simulink model "NIMBY"  (R2023a)
settings: Solver=VariableStepAuto  StartTime=0.0  StopTime=runtime  RelTol=1e-3
values from neighbouring files (symbols this model uses):
  DroneMass = 0.1    [NimbyCode.m]
  Dx = 1.5    [NimbyCode.m]
  Dy = 1.5    [NimbyCode.m]
  Dz = 2.5    [NimbyCode.m]
  escapeMargin = 1    [NimbyCode.m]
  Gravity = 9.81    [NimbyCode.m]
  InitialWPS = [InitialPosition; 0 0 -10]    [NimbyCode.m]
  Ix = 0    [NimbyCode.m]
  Iy = 0    [NimbyCode.m]
  Iz = 0    [NimbyCode.m]
  Nx = 1.25*10    (= 12.5)    [NimbyCode.m]
  Ny = 1.25*10    (= 12.5)    [NimbyCode.m]
  Nz = 1.25*14.4947065605712    (= 18.1183832007)    [NimbyCode.m]
  obstacleHeight = 15    [NimbyCode.m]
  obstaclePos = [5 5 0;5 25 0; 25 25 0; 25 5 0]    [NimbyCode.m]
  obstacleWidth = 5    [NimbyCode.m]
  Px = 6    [NimbyCode.m]
  Py = 6    [NimbyCode.m]
  Pz = 6.5    [NimbyCode.m]
  UAVSampleTime = 0.01    [NimbyCode.m]
libraries: slpidlib x6, dspsrcs4 x4, uavsimlib x4, robotcorelib x2, uavalgslib x2
settings Model: PacingRate=1000  Creator=JoshJ  LastModifiedBy=JoshJ
settings DebuggingCC: ParameterOverflowMsg=none  ParameterPrecisionLossMsg=none

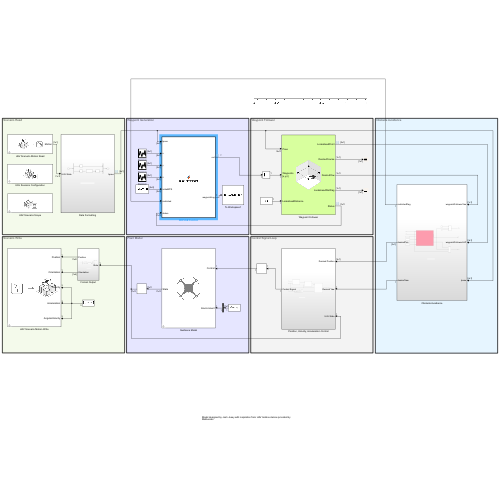
[thumbnail: Simulink's stored preview of the top-level diagram]
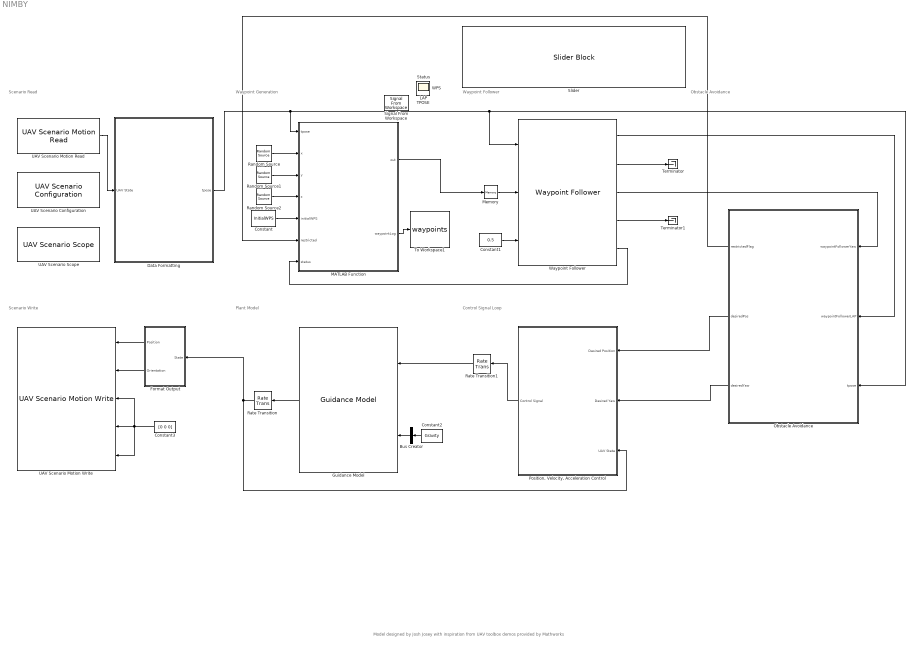
== system NIMBY ==
  note: Model designed by Josh Josey with inspiration from UAV toolbox demos provided by Mathworks
  note: Obstacle Avoidance
  note: Control Signal Loop
  note: Waypoint Follower
  note: Scenario Read
  note: Plant Model
  note: Scenario Write
  note: Waypoint Generation
  Bus Creator : BusCreator  Inputs=1  OutDataTypeStr=Bus: uavGuidanceEnvironmentBus  NonVirtualBus=on
      settings: InheritFromInputs=off
  Constant : Constant  Value=InitialWPS
  Constant1 : Constant  Value=0.5
  Constant2 : Constant  Value=Gravity  OutDataTypeStr=double
  Constant3 : Constant  Value=[0 0 0]
  Data Formatting : Subsystem
  Format Output : Subsystem
  Guidance Model : uavalgslib/Guidance Model  ModelType=MultirotorGuidance  SpecifiedDataType=double  SimulateUsing=Code generation  InitialWorldPositionMultirotor=InitialPosition'  InitialWorldVelocityMultirotor=[0; 0; 0]  InitialEulerZYXMultirotor=[0; 0; 0]  InitialBodyAngularRateRPYMultirotor=[0; 0; 0]  InitialThrustMultirotor=0  InitialNorthFixedWing=0  InitialEastFixedWing=0  InitialHeightFixedWing=0  InitialAirSpeedFixedWing=0  InitialHeadingAngleFixedWing=0  InitialFlightPathAngleFixedWing=0  InitialRollAngleFixedWing=0  InitialRollAngleRateFixedWing=0  PDRollMultirotor=[3402.97,116.67]  PDPitchMultirotor=[3402.97, 116.67]  PYawRateMultirotor=1950  PThrustMultirotor=3900  MassMultirotor=0.1  PHeightFixedWing=3.9  PHeadingAngleFixedWing=3.9  PFlightPathAngleFixedWing=39  PDRollFixedWing=[3402.97, 116.67]  PAirSpeedFixedWing=1  FlightPathAngleLimitsFixedWing=[-pi/2, pi/2]  StateBusName='uavGuidanceStateBus'  ControlBusName='uavGuidanceControlBus'  EnvironmentBusName='uavGuidanceEnvironmentBus'  DataType=double
  MATLAB Function : MATLAB Function  TreatAsAtomicUnit=on  SystemSampleTime=UAVSampleTime
  Memory : Memory
  Obstacle Avoidance : Subsystem
  "Position, Velocity, Acceleration Control" : Subsystem
  Random Source : dspsrcs4/Random Source  SrcType=Uniform  NormMethod=Ziggurat  CltLength=12  MinVal=0  MaxVal=30  MeanVal=0  VarVal=1  RepMode=Not repeatable  rawSeed=1  IsInherit=off  SampMode=Discrete  SampTime=UAVSampleTime  SampFrame=2  DataType=Double  OutComplex=Real  OutputFrames=off
  Random Source1 : dspsrcs4/Random Source  SrcType=Uniform  NormMethod=Ziggurat  CltLength=12  MinVal=0  MaxVal=30  MeanVal=0  VarVal=1  RepMode=Not repeatable  rawSeed=1  IsInherit=off  SampMode=Discrete  SampTime=UAVSampleTime  SampFrame=2  DataType=Double  OutComplex=Real  OutputFrames=off
  Random Source2 : dspsrcs4/Random Source  SrcType=Uniform  NormMethod=Ziggurat  CltLength=12  MinVal=5  MaxVal=20  MeanVal=0  VarVal=1  RepMode=Not repeatable  rawSeed=1  IsInherit=off  SampMode=Discrete  SampTime=UAVSampleTime  SampFrame=2  DataType=Double  OutComplex=Real  OutputFrames=off
  Rate Transition : RateTransition  OutPortSampleTime=UAVSampleTime
  Rate Transition1 : RateTransition  OutPortSampleTime=UAVSampleTime
  Slider : SliderBlock  LabelPosition=Hide  ScaleMax=1  TickInterval=.2
  Terminator : Terminator
  Terminator1 : Terminator
  To Workspace1 : ToWorkspace  VariableName=waypoints  SampleTime=-1
  UAV Scenario Configuration : uavsimlib/UAV Scenario Configuration  Priority=-1  UAVScenarioObject=Scenario  SampleTime=0.1  UpdateParam=false  SensorMotionBusName='SensorMotionBus'  PlatformMotionBusName='PlatformMotionBus'  ScenarioMotionBusName='ScenarioMotionBus'  ScenarioMotionSignalName='ScenarioMotions'
  UAV Scenario Motion Read : uavsimlib/UAV Scenario Motion Read  Priority=1  EntityName='UAV'  ReferenceFrame=NED
  UAV Scenario Motion Write : uavsimlib/UAV Scenario Motion Write  Priority=0  PlatName='UAV'  ReferenceFrame=NED
  UAV Scenario Scope : uavsimlib/UAV Scenario Scope  Priority=1  SensorNameTable={}  SampleTime=0.1
  Waypoint Follower : uavalgslib/Waypoint Follower  UAVType=multirotor  StartFrom=first  TransitionRadiusSource=internal  TransitionRadius=.1  MinLookaheadDistance=.2  YawInput=off  ShowCrossTrackErrorOutput=off  ShowStatusOutput=on  SimulateUsing=Code generation
  LAP : Scope
  Signal From Workspace : dspsrcs4/Signal From Workspace  IOType=siggen  X=1:10  Ts=1  nsamps=1  OutputAfterFinalValue=Setting to zero  ignoreOrWarnInputAndFrameLengths=off  OutputFrames=on
      settings: LibrarySourceBlock=|
      | dspgenerators/Signal From
      | Workspace
  Status : Scope
  TPOSE : Scope
  WPS : Scope
  wires:
  UAV Scenario Motion Read/1 -> Data Formatting/1(UAV State)
  Data Formatting/1(tpose) -> MATLAB Function/1(tpose), Obstacle Avoidance/3(tpose), Waypoint Follower/1
  Constant1/1 -> Waypoint Follower/3
  Waypoint Follower/2 -> Terminator/1
  Waypoint Follower/4 -> Terminator1/1
  Guidance Model/1 -> Rate Transition/1
  Rate Transition/1 -> Format Output/1(State), "Position, Velocity, Acceleration Control"/3(UAV State)
  Bus Creator/1 -> Guidance Model/2
  Constant2/1 -> Bus Creator/1
  Rate Transition1/1 -> Guidance Model/1
  Constant3/1 -> UAV Scenario Motion Write/5, UAV Scenario Motion Write/3, UAV Scenario Motion Write/4
  Format Output/2(Orientation) -> UAV Scenario Motion Write/2
  Format Output/1(Position) -> UAV Scenario Motion Write/1
  Waypoint Follower/5 -> MATLAB Function/7(status)
  Memory/1 -> Waypoint Follower/2
  MATLAB Function/1(out) -> Memory/1
  "Position, Velocity, Acceleration Control"/1(Control Signal) -> Rate Transition1/1
  Waypoint Follower/1 -> Obstacle Avoidance/2(waypointFollowerLAP)
  Waypoint Follower/3 -> Obstacle Avoidance/1(waypointFollowerYaw)
  Obstacle Avoidance/1(restrictedFlag) -> MATLAB Function/6(restricted)
  Obstacle Avoidance/2(desiredPos) -> "Position, Velocity, Acceleration Control"/1(Desired Position)
  Obstacle Avoidance/3(desiredYaw) -> "Position, Velocity, Acceleration Control"/2(Desired Yaw)
  MATLAB Function/2(waypointLog) -> To Workspace1/1
  Constant/1 -> MATLAB Function/5(initialWPS)
  Random Source2/1 -> MATLAB Function/4(z)
  Random Source1/1 -> MATLAB Function/3(y)
  Random Source/1 -> MATLAB Function/2(x)

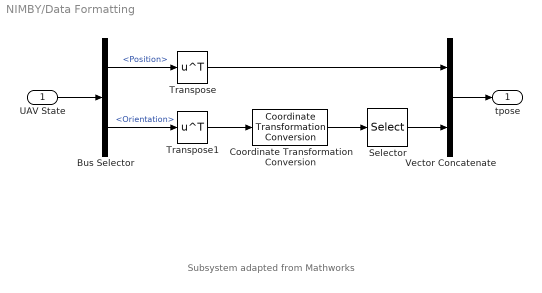
== system NIMBY/Data Formatting ==
  note: Subsystem adapted from Mathworks
  UAV State : Inport
  Bus Selector : BusSelector  OutputSignals=Position,Orientation
  Coordinate Transformation Conversion : robotcorelib/Coordinate Transformation Conversion  InputRepresentation=Quaternion  InputEulerSequence=ZYX  ShowTrVecInputPort=on  OutputRepresentation=Euler Angles  OutputEulerSequence=ZYX  ShowTrVecOutputPort=on  SimulateUsing=Interpreted execution
      settings: LibrarySourceBlock=navlib/Utilities/Coordinate Transformation Conversion
  Selector : Selector  InputPortWidth=3  IndexOptions=Index vector (dialog)  Indices=[1]  OutputSizes=1
  Transpose : Math  Operator=transpose
  Transpose1 : Math  Operator=transpose
  Vector Concatenate : Concatenate
  tpose : Outport
  wires:
  UAV State/1 -> Bus Selector/1
  Transpose1/1 -> Coordinate Transformation Conversion/1
  Bus Selector/1 -> Transpose/1  "<Position>"
  Bus Selector/2 -> Transpose1/1  "<Orientation>"
  Vector Concatenate/1 -> tpose/1
  Transpose/1 -> Vector Concatenate/1
  Coordinate Transformation Conversion/1 -> Selector/1
  Selector/1 -> Vector Concatenate/2

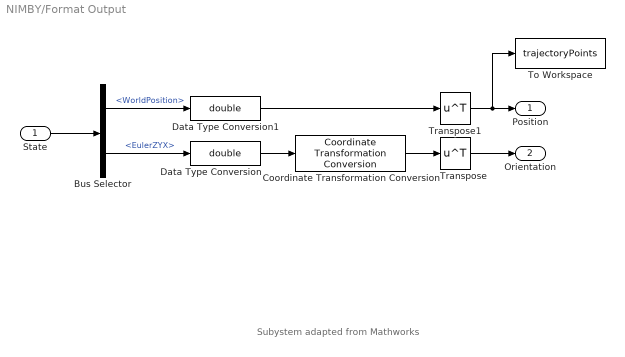
== system NIMBY/Format Output ==
  note: Subystem adapted from Mathworks
  State : Inport
  Bus Selector : BusSelector  OutputSignals=WorldPosition,EulerZYX
  Coordinate Transformation Conversion : robotcorelib/Coordinate Transformation Conversion  InputRepresentation=Euler Angles  InputEulerSequence=ZYX  ShowTrVecInputPort=on  OutputRepresentation=Quaternion  OutputEulerSequence=ZYX  ShowTrVecOutputPort=on  SimulateUsing=Code generation
      settings: LibrarySourceBlock=navlib/Utilities/Coordinate Transformation Conversion
  Data Type Conversion : DataTypeConversion  OutDataTypeStr=double  SaturateOnIntegerOverflow=off  RndMeth=Floor
  Data Type Conversion1 : DataTypeConversion  OutDataTypeStr=double  SaturateOnIntegerOverflow=off  RndMeth=Floor
  To Workspace : ToWorkspace  VariableName=trajectoryPoints  SampleTime=-1
  Transpose : Math  Operator=transpose
  Transpose1 : Math  Operator=transpose
  Position : Outport
  Orientation : Outport  Port=2
  wires:
  State/1 -> Bus Selector/1
  Bus Selector/1 -> Data Type Conversion1/1  "<WorldPosition>"
  Bus Selector/2 -> Data Type Conversion/1  "<EulerZYX>"
  Data Type Conversion/1 -> Coordinate Transformation Conversion/1
  Transpose/1 -> Orientation/1
  Coordinate Transformation Conversion/1 -> Transpose/1
  Data Type Conversion1/1 -> Transpose1/1
  Transpose1/1 -> To Workspace/1, Position/1

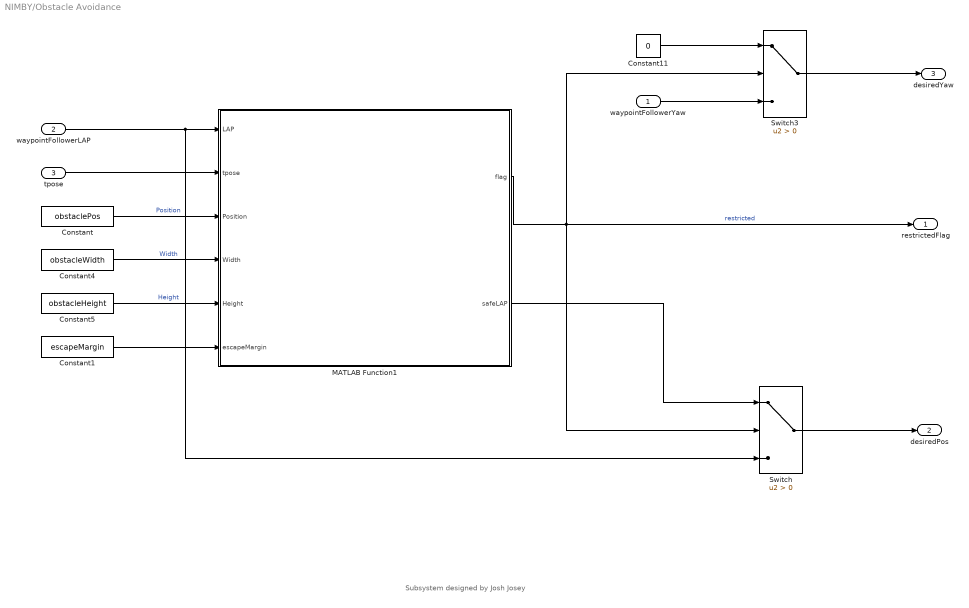
== system NIMBY/Obstacle Avoidance ==
  note: Subsystem designed by Josh Josey
  waypointFollowerYaw : Inport
  waypointFollowerLAP : Inport  Port=2
  tpose : Inport  Port=3
  Constant : Constant  Value=obstaclePos
  Constant1 : Constant  Value=escapeMargin
  Constant11 : Constant  Value=0
  Constant4 : Constant  Value=obstacleWidth
  Constant5 : Constant  Value=obstacleHeight
  MATLAB Function1 : MATLAB Function  TreatAsAtomicUnit=on
  Switch : Switch  Criteria=u2 > Threshold  SaturateOnIntegerOverflow=off  InputSameDT=off
  Switch3 : Switch  Criteria=u2 > Threshold  SaturateOnIntegerOverflow=off  InputSameDT=off
  restrictedFlag : Outport
  desiredPos : Outport  Port=2
  desiredYaw : Outport  Port=3
  wires:
  tpose/1 -> MATLAB Function1/2(tpose)
  Constant4/1 -> MATLAB Function1/4(Width)  "Width"
  Constant11/1 -> Switch3/1
  MATLAB Function1/1(flag) -> Switch3/2, Switch/2, restrictedFlag/1  "restricted"
  Constant5/1 -> MATLAB Function1/5(Height)  "Height"
  Constant/1 -> MATLAB Function1/3(Position)  "Position"
  Switch3/1 -> desiredYaw/1
  waypointFollowerLAP/1 -> Switch/3, MATLAB Function1/1(LAP)
  Switch/1 -> desiredPos/1
  waypointFollowerYaw/1 -> Switch3/3
  MATLAB Function1/2(safeLAP) -> Switch/1
  Constant1/1 -> MATLAB Function1/6(escapeMargin)

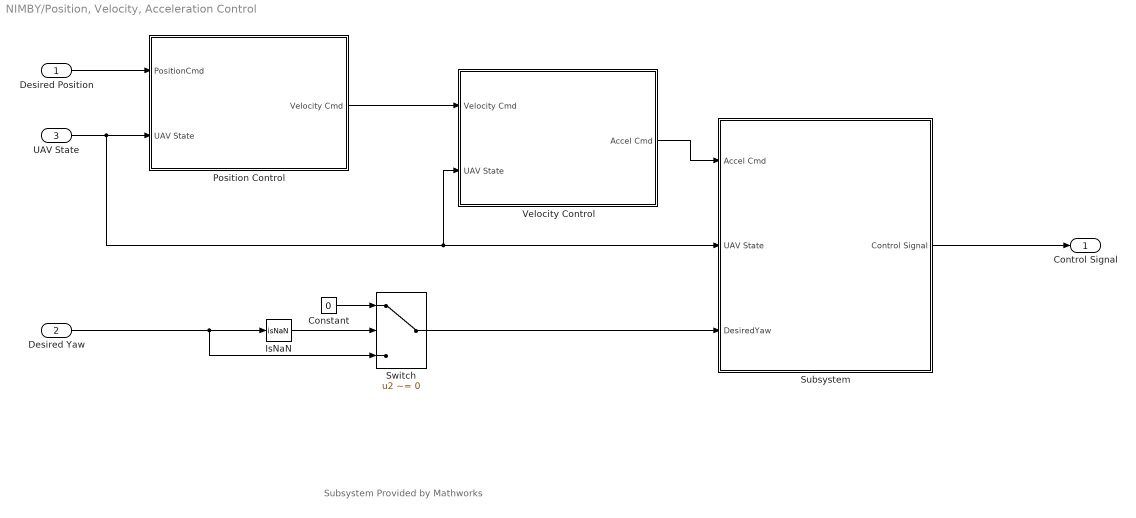
== system NIMBY/Position, Velocity, Acceleration Control ==
  note: Subsystem Provided by Mathworks
  Desired Position : Inport
  Desired Yaw : Inport  Port=2
  UAV State : Inport  Port=3
  Constant : Constant  Value=0  OutDataTypeStr=Inherit: Inherit via back propagation
  IsNaN : RelationalOperator  Operator=isNaN  OutDataTypeStr=boolean  RndMeth=Simplest  InputSameDT=off
  Position Control : Subsystem
  Subsystem : Subsystem
  Switch : Switch  Criteria=u2 ~= 0  SaturateOnIntegerOverflow=off  InputSameDT=off
  Velocity Control : Subsystem
  Control Signal : Outport
  wires:
  Desired Yaw/1 -> Switch/3, IsNaN/1
  UAV State/1 -> Subsystem/2(UAV State), Velocity Control/2(UAV State), Position Control/2(UAV State)
  Desired Position/1 -> Position Control/1(PositionCmd)
  Position Control/1(Velocity Cmd) -> Velocity Control/1(Velocity Cmd)
  Subsystem/1(Control Signal) -> Control Signal/1
  Velocity Control/1(Accel Cmd) -> Subsystem/1(Accel Cmd)
  IsNaN/1 -> Switch/2
  Constant/1 -> Switch/1
  Switch/1 -> Subsystem/3(DesiredYaw)

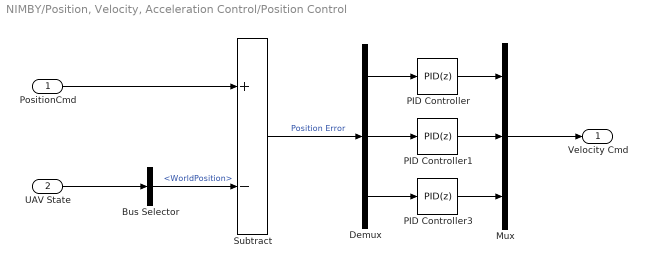
== system NIMBY/Position, Velocity, Acceleration Control/Position Control ==
  PositionCmd : Inport
  UAV State : Inport  Port=2
  Bus Selector : BusSelector  OutputSignals=WorldPosition
  Demux : Demux  Outputs=3
  Mux : Mux  Inputs=3
  PID Controller : slpidlib/PID Controller  Controller=PID  Form=Parallel  TimeDomain=Discrete-time  UseExternalTs=off  SampleTime=-1  IntegratorMethod=Forward Euler  FilterMethod=Forward Euler  ControllerParametersSource=internal  P=Px  I=Ix  UseKiTs=off  D=Dx  N=Nx  UseFilter=on  TunerSelectOption=Transfer Function Based (PID Tuner App)  InitialConditionSource=internal  InitialConditionForIntegrator=0  InitialConditionForFilter=0  DifferentiatorICPrevScaledInput=0  ExternalReset=none  TrackingMode=off  Kt=1  LimitOutput=on  SatLimitsSource=internal  UpperSaturationLimit=3  LowerSaturationLimit=-3  LinearizeAsGain=on  AntiWindupMode=clamping  Kb=1  LimitIntegrator=off  UpperIntegratorSaturationLimit=inf  LowerIntegratorSaturationLimit=-inf  POutMin=[]  POutMax=[]  IOutMin=[]  IOutMax=[]  DOutMin=[]  DOutMax=[]  NOutMin=[]  NOutMax=[]  SumOutMin=[]  SumOutMax=[]  SaturationOutMin=[]  SaturationOutMax=[]  PParamMin=[]  PParamMax=[]  IParamMin=[]  IParamMax=[]  DParamMin=[]  DParamMax=[]  NParamMin=[]  NParamMax=[]  KbParamMin=[]  KbParamMax=[]  KtParamMin=[]  KtParamMax=[]  KbOutMin=[]  KbOutMax=[]  KtOutMin=[]  KtOutMax=[]  IntegratorOutMin=[]  IntegratorOutMax=[]  FilterOutMin=[]  FilterOutMax=[]  SumI1OutMin=[]  SumI1OutMax=[]  SumI2OutMin=[]  SumI2OutMax=[]  SumI3OutMin=[]  SumI3OutMax=[]  SumI4OutMin=[]  SumI4OutMax=[]  SumDOutMin=[]  SumDOutMax=[]  DifferentiatorOutMin=[]  DifferentiatorOutMax=[]  FilterDiffOutCoefMin=[]  FilterDiffOutCoefMax=[]  ReciprocalOutMin=[]  ReciprocalOutMax=[]  SumDenOutMin=[]  SumDenOutMax=[]  SumNumOutMin=[]  SumNumOutMax=[]  DivideOutMin=[]  DivideOutMax=[]  UdiffTsProdOutMin=[]  UdiffTsProdOutMax=[]  NTsProdOutMin=[]  NTsProdOutMax=[]  UintegralTsProdOutMin=[]  UintegralTsProdOutMax=[]  UngainTsProdOutMin=[]  UngainTsProdOutMax=[]  ClampingZeroOutDataTypeStr=Inherit: Inherit via back propagation  ClampingZeroOutMin=[]  ClampingZeroOutMax=[]  FilterDenConstantOutDataTypeStr=Inherit: Inherit via back propagation  FilterDenConstantOutMin=[]  FilterDenConstantOutMax=[]  PCopyOutDataTypeStr=Inherit: Inherit via back propagation  PCopyOutMin=[]  PCopyOutMax=[]  NCopyOutDataTypeStr=Inherit: Inherit via back propagation  NCopyOutMin=[]  NCopyOutMax=[]  IntegratorContinuousStateAttributes=''  IntegratorStateMustResolveToSignalObject=off  IntegratorRTWStateStorageClass=Auto  FilterContinuousStateAttributes=''  FilterStateMustResolveToSignalObject=off  FilterRTWStateStorageClass=Auto  ParallelPVariant=InternalParameters  IdealPVariant=Disabled  IVariant=InternalParameters  DVariant=InternalParameters  IntegratorVariant=Discrete  SatVariant=Enabled  AWVariant=DiscClampingParallel  PCopyVariant=Disabled  TRVariant=Disabled  FdbkBlocksVariant=Forward  IdealPFdbkVariant=Disabled  SatFdbkVariant=Disabled  DerivativeFilterVariant=ForwardEulerFilter  NVariant=InternalParameters  NCopyVariant=Disabled  FilterICVariant=InternalICsFilter  IntegratorICVariant=InternalICs  ExternalResetVariant=Disabled  TRSumVariant=Passthrough  SumFdbkVariant=Disabled  SumVariant=Sum_PID  TsampFilterVariant=InternalTs  TsampNgainVariant=Passthrough  TsampIntegralVariant=Disabled_SignalSpec  ExternalSaturationOutDataTypeStr=Inherit: Same as second input
  PID Controller1 : slpidlib/PID Controller  Controller=PID  Form=Parallel  TimeDomain=Discrete-time  UseExternalTs=off  SampleTime=-1  IntegratorMethod=Forward Euler  FilterMethod=Forward Euler  ControllerParametersSource=internal  P=Py  I=Iy  UseKiTs=off  D=Dy  N=Ny  UseFilter=on  TunerSelectOption=Transfer Function Based (PID Tuner App)  InitialConditionSource=internal  InitialConditionForIntegrator=0  InitialConditionForFilter=0  DifferentiatorICPrevScaledInput=0  ExternalReset=none  TrackingMode=off  Kt=1  LimitOutput=on  SatLimitsSource=internal  UpperSaturationLimit=3  LowerSaturationLimit=-3  LinearizeAsGain=on  AntiWindupMode=clamping  Kb=1  LimitIntegrator=off  UpperIntegratorSaturationLimit=inf  LowerIntegratorSaturationLimit=-inf  POutMin=[]  POutMax=[]  IOutMin=[]  IOutMax=[]  DOutMin=[]  DOutMax=[]  NOutMin=[]  NOutMax=[]  SumOutMin=[]  SumOutMax=[]  SaturationOutMin=[]  SaturationOutMax=[]  PParamMin=[]  PParamMax=[]  IParamMin=[]  IParamMax=[]  DParamMin=[]  DParamMax=[]  NParamMin=[]  NParamMax=[]  KbParamMin=[]  KbParamMax=[]  KtParamMin=[]  KtParamMax=[]  KbOutMin=[]  KbOutMax=[]  KtOutMin=[]  KtOutMax=[]  IntegratorOutMin=[]  IntegratorOutMax=[]  FilterOutMin=[]  FilterOutMax=[]  SumI1OutMin=[]  SumI1OutMax=[]  SumI2OutMin=[]  SumI2OutMax=[]  SumI3OutMin=[]  SumI3OutMax=[]  SumI4OutMin=[]  SumI4OutMax=[]  SumDOutMin=[]  SumDOutMax=[]  DifferentiatorOutMin=[]  DifferentiatorOutMax=[]  FilterDiffOutCoefMin=[]  FilterDiffOutCoefMax=[]  ReciprocalOutMin=[]  ReciprocalOutMax=[]  SumDenOutMin=[]  SumDenOutMax=[]  SumNumOutMin=[]  SumNumOutMax=[]  DivideOutMin=[]  DivideOutMax=[]  UdiffTsProdOutMin=[]  UdiffTsProdOutMax=[]  NTsProdOutMin=[]  NTsProdOutMax=[]  UintegralTsProdOutMin=[]  UintegralTsProdOutMax=[]  UngainTsProdOutMin=[]  UngainTsProdOutMax=[]  ClampingZeroOutDataTypeStr=Inherit: Inherit via back propagation  ClampingZeroOutMin=[]  ClampingZeroOutMax=[]  FilterDenConstantOutDataTypeStr=Inherit: Inherit via back propagation  FilterDenConstantOutMin=[]  FilterDenConstantOutMax=[]  PCopyOutDataTypeStr=Inherit: Inherit via back propagation  PCopyOutMin=[]  PCopyOutMax=[]  NCopyOutDataTypeStr=Inherit: Inherit via back propagation  NCopyOutMin=[]  NCopyOutMax=[]  IntegratorContinuousStateAttributes=''  IntegratorStateMustResolveToSignalObject=off  IntegratorRTWStateStorageClass=Auto  FilterContinuousStateAttributes=''  FilterStateMustResolveToSignalObject=off  FilterRTWStateStorageClass=Auto  ParallelPVariant=InternalParameters  IdealPVariant=Disabled  IVariant=InternalParameters  DVariant=InternalParameters  IntegratorVariant=Discrete  SatVariant=Enabled  AWVariant=DiscClampingParallel  PCopyVariant=Disabled  TRVariant=Disabled  FdbkBlocksVariant=Forward  IdealPFdbkVariant=Disabled  SatFdbkVariant=Disabled  DerivativeFilterVariant=ForwardEulerFilter  NVariant=InternalParameters  NCopyVariant=Disabled  FilterICVariant=InternalICsFilter  IntegratorICVariant=InternalICs  ExternalResetVariant=Disabled  TRSumVariant=Passthrough  SumFdbkVariant=Disabled  SumVariant=Sum_PID  TsampFilterVariant=InternalTs  TsampNgainVariant=Passthrough  TsampIntegralVariant=Disabled_SignalSpec  ExternalSaturationOutDataTypeStr=Inherit: Same as second input
  PID Controller3 : slpidlib/PID Controller  Controller=PID  Form=Parallel  TimeDomain=Discrete-time  UseExternalTs=off  SampleTime=-1  IntegratorMethod=Forward Euler  FilterMethod=Forward Euler  ControllerParametersSource=internal  P=Pz  I=Iz  UseKiTs=off  D=Dz  N=Nz  UseFilter=on  TunerSelectOption=Transfer Function Based (PID Tuner App)  InitialConditionSource=internal  InitialConditionForIntegrator=0  InitialConditionForFilter=0  DifferentiatorICPrevScaledInput=0  ExternalReset=none  TrackingMode=off  Kt=1  LimitOutput=on  SatLimitsSource=internal  UpperSaturationLimit=3  LowerSaturationLimit=-3  LinearizeAsGain=on  AntiWindupMode=clamping  Kb=1  LimitIntegrator=off  UpperIntegratorSaturationLimit=inf  LowerIntegratorSaturationLimit=-inf  POutMin=[]  POutMax=[]  IOutMin=[]  IOutMax=[]  DOutMin=[]  DOutMax=[]  NOutMin=[]  NOutMax=[]  SumOutMin=[]  SumOutMax=[]  SaturationOutMin=[]  SaturationOutMax=[]  PParamMin=[]  PParamMax=[]  IParamMin=[]  IParamMax=[]  DParamMin=[]  DParamMax=[]  NParamMin=[]  NParamMax=[]  KbParamMin=[]  KbParamMax=[]  KtParamMin=[]  KtParamMax=[]  KbOutMin=[]  KbOutMax=[]  KtOutMin=[]  KtOutMax=[]  IntegratorOutMin=[]  IntegratorOutMax=[]  FilterOutMin=[]  FilterOutMax=[]  SumI1OutMin=[]  SumI1OutMax=[]  SumI2OutMin=[]  SumI2OutMax=[]  SumI3OutMin=[]  SumI3OutMax=[]  SumI4OutMin=[]  SumI4OutMax=[]  SumDOutMin=[]  SumDOutMax=[]  DifferentiatorOutMin=[]  DifferentiatorOutMax=[]  FilterDiffOutCoefMin=[]  FilterDiffOutCoefMax=[]  ReciprocalOutMin=[]  ReciprocalOutMax=[]  SumDenOutMin=[]  SumDenOutMax=[]  SumNumOutMin=[]  SumNumOutMax=[]  DivideOutMin=[]  DivideOutMax=[]  UdiffTsProdOutMin=[]  UdiffTsProdOutMax=[]  NTsProdOutMin=[]  NTsProdOutMax=[]  UintegralTsProdOutMin=[]  UintegralTsProdOutMax=[]  UngainTsProdOutMin=[]  UngainTsProdOutMax=[]  ClampingZeroOutDataTypeStr=Inherit: Inherit via back propagation  ClampingZeroOutMin=[]  ClampingZeroOutMax=[]  FilterDenConstantOutDataTypeStr=Inherit: Inherit via back propagation  FilterDenConstantOutMin=[]  FilterDenConstantOutMax=[]  PCopyOutDataTypeStr=Inherit: Inherit via back propagation  PCopyOutMin=[]  PCopyOutMax=[]  NCopyOutDataTypeStr=Inherit: Inherit via back propagation  NCopyOutMin=[]  NCopyOutMax=[]  IntegratorContinuousStateAttributes=''  IntegratorStateMustResolveToSignalObject=off  IntegratorRTWStateStorageClass=Auto  FilterContinuousStateAttributes=''  FilterStateMustResolveToSignalObject=off  FilterRTWStateStorageClass=Auto  ParallelPVariant=InternalParameters  IdealPVariant=Disabled  IVariant=InternalParameters  DVariant=InternalParameters  IntegratorVariant=Discrete  SatVariant=Enabled  AWVariant=DiscClampingParallel  PCopyVariant=Disabled  TRVariant=Disabled  FdbkBlocksVariant=Forward  IdealPFdbkVariant=Disabled  SatFdbkVariant=Disabled  DerivativeFilterVariant=ForwardEulerFilter  NVariant=InternalParameters  NCopyVariant=Disabled  FilterICVariant=InternalICsFilter  IntegratorICVariant=InternalICs  ExternalResetVariant=Disabled  TRSumVariant=Passthrough  SumFdbkVariant=Disabled  SumVariant=Sum_PID  TsampFilterVariant=InternalTs  TsampNgainVariant=Passthrough  TsampIntegralVariant=Disabled_SignalSpec  ExternalSaturationOutDataTypeStr=Inherit: Same as second input
  Subtract : Sum  Inputs=+-
  Velocity Cmd : Outport
  wires:
  UAV State/1 -> Bus Selector/1
  PositionCmd/1 -> Subtract/1
  Bus Selector/1 -> Subtract/2  "<WorldPosition>"
  Subtract/1 -> Demux/1  "Position Error"
  Demux/1 -> PID Controller/1
  Demux/2 -> PID Controller1/1
  Demux/3 -> PID Controller3/1
  PID Controller3/1 -> Mux/3
  Mux/1 -> Velocity Cmd/1
  PID Controller1/1 -> Mux/2
  PID Controller/1 -> Mux/1

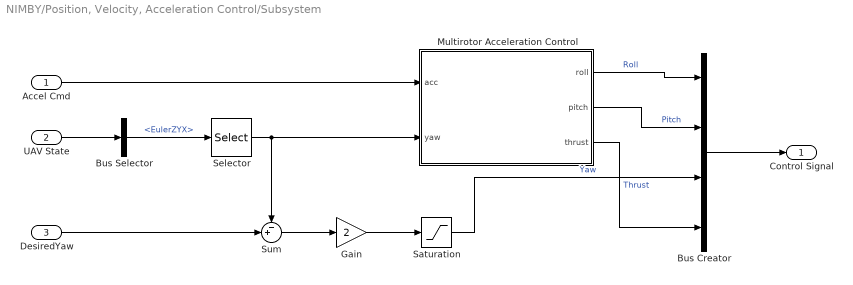
== system NIMBY/Position, Velocity, Acceleration Control/Subsystem ==
  Accel Cmd : Inport
  UAV State : Inport  Port=2
  DesiredYaw : Inport  Port=3
  Bus Creator : BusCreator  Inputs=4  OutDataTypeStr=Bus: uavGuidanceControlBus  NonVirtualBus=on
      settings: InheritFromInputs=off
  Bus Selector : BusSelector  OutputSignals=EulerZYX
  Gain : Gain  Gain=2
  Multirotor Acceleration Control : MATLAB Function  TreatAsAtomicUnit=on
  Saturation : Saturate
  Selector : Selector  InputPortWidth=3  IndexOptions=Index vector (dialog)  Indices=1  OutputSizes=1
  Sum : Sum  Inputs=-+|
  Control Signal : Outport
  wires:
  Multirotor Acceleration Control/2(pitch) -> Bus Creator/2  "Pitch"
  Multirotor Acceleration Control/1(roll) -> Bus Creator/1  "Roll"
  Bus Creator/1 -> Control Signal/1
  Multirotor Acceleration Control/3(thrust) -> Bus Creator/4  "Thrust"
  Accel Cmd/1 -> Multirotor Acceleration Control/1(acc)
  UAV State/1 -> Bus Selector/1
  Bus Selector/1 -> Selector/1  "<EulerZYX>"
  Selector/1 -> Sum/1, Multirotor Acceleration Control/2(yaw)
  DesiredYaw/1 -> Sum/2
  Sum/1 -> Gain/1
  Gain/1 -> Saturation/1
  Saturation/1 -> Bus Creator/3  "Yaw"

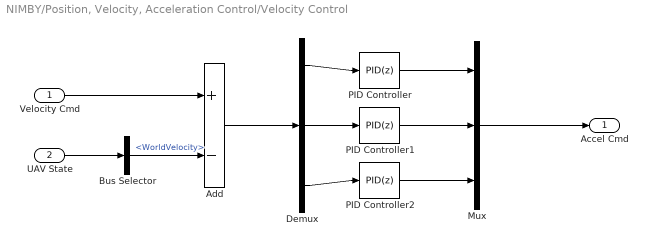
== system NIMBY/Position, Velocity, Acceleration Control/Velocity Control ==
  Velocity Cmd : Inport
  UAV State : Inport  Port=2
  Add : Sum  Inputs=+-
  Bus Selector : BusSelector  OutputSignals=WorldVelocity
  Demux : Demux  Outputs=3
  Mux : Mux  Inputs=3
  PID Controller : slpidlib/PID Controller  Controller=PID  Form=Parallel  TimeDomain=Discrete-time  UseExternalTs=off  SampleTime=-1  IntegratorMethod=Forward Euler  FilterMethod=Forward Euler  ControllerParametersSource=internal  P=Px  I=Ix  UseKiTs=off  D=Dx  N=Nx  UseFilter=on  TunerSelectOption=Transfer Function Based (PID Tuner App)  InitialConditionSource=internal  InitialConditionForIntegrator=0  InitialConditionForFilter=0  DifferentiatorICPrevScaledInput=0  ExternalReset=none  TrackingMode=off  Kt=1  LimitOutput=on  SatLimitsSource=internal  UpperSaturationLimit=3  LowerSaturationLimit=-3  LinearizeAsGain=on  AntiWindupMode=clamping  Kb=1  LimitIntegrator=off  UpperIntegratorSaturationLimit=inf  LowerIntegratorSaturationLimit=-inf  POutMin=[]  POutMax=[]  IOutMin=[]  IOutMax=[]  DOutMin=[]  DOutMax=[]  NOutMin=[]  NOutMax=[]  SumOutMin=[]  SumOutMax=[]  SaturationOutMin=[]  SaturationOutMax=[]  PParamMin=[]  PParamMax=[]  IParamMin=[]  IParamMax=[]  DParamMin=[]  DParamMax=[]  NParamMin=[]  NParamMax=[]  KbParamMin=[]  KbParamMax=[]  KtParamMin=[]  KtParamMax=[]  KbOutMin=[]  KbOutMax=[]  KtOutMin=[]  KtOutMax=[]  IntegratorOutMin=[]  IntegratorOutMax=[]  FilterOutMin=[]  FilterOutMax=[]  SumI1OutMin=[]  SumI1OutMax=[]  SumI2OutMin=[]  SumI2OutMax=[]  SumI3OutMin=[]  SumI3OutMax=[]  SumI4OutMin=[]  SumI4OutMax=[]  SumDOutMin=[]  SumDOutMax=[]  DifferentiatorOutMin=[]  DifferentiatorOutMax=[]  FilterDiffOutCoefMin=[]  FilterDiffOutCoefMax=[]  ReciprocalOutMin=[]  ReciprocalOutMax=[]  SumDenOutMin=[]  SumDenOutMax=[]  SumNumOutMin=[]  SumNumOutMax=[]  DivideOutMin=[]  DivideOutMax=[]  UdiffTsProdOutMin=[]  UdiffTsProdOutMax=[]  NTsProdOutMin=[]  NTsProdOutMax=[]  UintegralTsProdOutMin=[]  UintegralTsProdOutMax=[]  UngainTsProdOutMin=[]  UngainTsProdOutMax=[]  ClampingZeroOutDataTypeStr=Inherit: Inherit via back propagation  ClampingZeroOutMin=[]  ClampingZeroOutMax=[]  FilterDenConstantOutDataTypeStr=Inherit: Inherit via back propagation  FilterDenConstantOutMin=[]  FilterDenConstantOutMax=[]  PCopyOutDataTypeStr=Inherit: Inherit via back propagation  PCopyOutMin=[]  PCopyOutMax=[]  NCopyOutDataTypeStr=Inherit: Inherit via back propagation  NCopyOutMin=[]  NCopyOutMax=[]  IntegratorContinuousStateAttributes=''  IntegratorStateMustResolveToSignalObject=off  IntegratorRTWStateStorageClass=Auto  FilterContinuousStateAttributes=''  FilterStateMustResolveToSignalObject=off  FilterRTWStateStorageClass=Auto  ParallelPVariant=InternalParameters  IdealPVariant=Disabled  IVariant=InternalParameters  DVariant=InternalParameters  IntegratorVariant=Discrete  SatVariant=Enabled  AWVariant=DiscClampingParallel  PCopyVariant=Disabled  TRVariant=Disabled  FdbkBlocksVariant=Forward  IdealPFdbkVariant=Disabled  SatFdbkVariant=Disabled  DerivativeFilterVariant=ForwardEulerFilter  NVariant=InternalParameters  NCopyVariant=Disabled  FilterICVariant=InternalICsFilter  IntegratorICVariant=InternalICs  ExternalResetVariant=Disabled  TRSumVariant=Passthrough  SumFdbkVariant=Disabled  SumVariant=Sum_PID  TsampFilterVariant=InternalTs  TsampNgainVariant=Passthrough  TsampIntegralVariant=Disabled_SignalSpec  ExternalSaturationOutDataTypeStr=Inherit: Same as second input
  PID Controller1 : slpidlib/PID Controller  Controller=PID  Form=Parallel  TimeDomain=Discrete-time  UseExternalTs=off  SampleTime=-1  IntegratorMethod=Forward Euler  FilterMethod=Forward Euler  ControllerParametersSource=internal  P=Px  I=Ix  UseKiTs=off  D=Dx  N=Nx  UseFilter=on  TunerSelectOption=Transfer Function Based (PID Tuner App)  InitialConditionSource=internal  InitialConditionForIntegrator=0  InitialConditionForFilter=0  DifferentiatorICPrevScaledInput=0  ExternalReset=none  TrackingMode=off  Kt=1  LimitOutput=on  SatLimitsSource=internal  UpperSaturationLimit=3  LowerSaturationLimit=-3  LinearizeAsGain=on  AntiWindupMode=clamping  Kb=1  LimitIntegrator=off  UpperIntegratorSaturationLimit=inf  LowerIntegratorSaturationLimit=-inf  POutMin=[]  POutMax=[]  IOutMin=[]  IOutMax=[]  DOutMin=[]  DOutMax=[]  NOutMin=[]  NOutMax=[]  SumOutMin=[]  SumOutMax=[]  SaturationOutMin=[]  SaturationOutMax=[]  PParamMin=[]  PParamMax=[]  IParamMin=[]  IParamMax=[]  DParamMin=[]  DParamMax=[]  NParamMin=[]  NParamMax=[]  KbParamMin=[]  KbParamMax=[]  KtParamMin=[]  KtParamMax=[]  KbOutMin=[]  KbOutMax=[]  KtOutMin=[]  KtOutMax=[]  IntegratorOutMin=[]  IntegratorOutMax=[]  FilterOutMin=[]  FilterOutMax=[]  SumI1OutMin=[]  SumI1OutMax=[]  SumI2OutMin=[]  SumI2OutMax=[]  SumI3OutMin=[]  SumI3OutMax=[]  SumI4OutMin=[]  SumI4OutMax=[]  SumDOutMin=[]  SumDOutMax=[]  DifferentiatorOutMin=[]  DifferentiatorOutMax=[]  FilterDiffOutCoefMin=[]  FilterDiffOutCoefMax=[]  ReciprocalOutMin=[]  ReciprocalOutMax=[]  SumDenOutMin=[]  SumDenOutMax=[]  SumNumOutMin=[]  SumNumOutMax=[]  DivideOutMin=[]  DivideOutMax=[]  UdiffTsProdOutMin=[]  UdiffTsProdOutMax=[]  NTsProdOutMin=[]  NTsProdOutMax=[]  UintegralTsProdOutMin=[]  UintegralTsProdOutMax=[]  UngainTsProdOutMin=[]  UngainTsProdOutMax=[]  ClampingZeroOutDataTypeStr=Inherit: Inherit via back propagation  ClampingZeroOutMin=[]  ClampingZeroOutMax=[]  FilterDenConstantOutDataTypeStr=Inherit: Inherit via back propagation  FilterDenConstantOutMin=[]  FilterDenConstantOutMax=[]  PCopyOutDataTypeStr=Inherit: Inherit via back propagation  PCopyOutMin=[]  PCopyOutMax=[]  NCopyOutDataTypeStr=Inherit: Inherit via back propagation  NCopyOutMin=[]  NCopyOutMax=[]  IntegratorContinuousStateAttributes=''  IntegratorStateMustResolveToSignalObject=off  IntegratorRTWStateStorageClass=Auto  FilterContinuousStateAttributes=''  FilterStateMustResolveToSignalObject=off  FilterRTWStateStorageClass=Auto  ParallelPVariant=InternalParameters  IdealPVariant=Disabled  IVariant=InternalParameters  DVariant=InternalParameters  IntegratorVariant=Discrete  SatVariant=Enabled  AWVariant=DiscClampingParallel  PCopyVariant=Disabled  TRVariant=Disabled  FdbkBlocksVariant=Forward  IdealPFdbkVariant=Disabled  SatFdbkVariant=Disabled  DerivativeFilterVariant=ForwardEulerFilter  NVariant=InternalParameters  NCopyVariant=Disabled  FilterICVariant=InternalICsFilter  IntegratorICVariant=InternalICs  ExternalResetVariant=Disabled  TRSumVariant=Passthrough  SumFdbkVariant=Disabled  SumVariant=Sum_PID  TsampFilterVariant=InternalTs  TsampNgainVariant=Passthrough  TsampIntegralVariant=Disabled_SignalSpec  ExternalSaturationOutDataTypeStr=Inherit: Same as second input
  PID Controller2 : slpidlib/PID Controller  Controller=PID  Form=Parallel  TimeDomain=Discrete-time  UseExternalTs=off  SampleTime=-1  IntegratorMethod=Forward Euler  FilterMethod=Forward Euler  ControllerParametersSource=internal  P=Px  I=Ix  UseKiTs=off  D=Dx  N=Nx  UseFilter=on  TunerSelectOption=Transfer Function Based (PID Tuner App)  InitialConditionSource=internal  InitialConditionForIntegrator=0  InitialConditionForFilter=0  DifferentiatorICPrevScaledInput=0  ExternalReset=none  TrackingMode=off  Kt=1  LimitOutput=on  SatLimitsSource=internal  UpperSaturationLimit=3  LowerSaturationLimit=-3  LinearizeAsGain=on  AntiWindupMode=clamping  Kb=1  LimitIntegrator=off  UpperIntegratorSaturationLimit=inf  LowerIntegratorSaturationLimit=-inf  POutMin=[]  POutMax=[]  IOutMin=[]  IOutMax=[]  DOutMin=[]  DOutMax=[]  NOutMin=[]  NOutMax=[]  SumOutMin=[]  SumOutMax=[]  SaturationOutMin=[]  SaturationOutMax=[]  PParamMin=[]  PParamMax=[]  IParamMin=[]  IParamMax=[]  DParamMin=[]  DParamMax=[]  NParamMin=[]  NParamMax=[]  KbParamMin=[]  KbParamMax=[]  KtParamMin=[]  KtParamMax=[]  KbOutMin=[]  KbOutMax=[]  KtOutMin=[]  KtOutMax=[]  IntegratorOutMin=[]  IntegratorOutMax=[]  FilterOutMin=[]  FilterOutMax=[]  SumI1OutMin=[]  SumI1OutMax=[]  SumI2OutMin=[]  SumI2OutMax=[]  SumI3OutMin=[]  SumI3OutMax=[]  SumI4OutMin=[]  SumI4OutMax=[]  SumDOutMin=[]  SumDOutMax=[]  DifferentiatorOutMin=[]  DifferentiatorOutMax=[]  FilterDiffOutCoefMin=[]  FilterDiffOutCoefMax=[]  ReciprocalOutMin=[]  ReciprocalOutMax=[]  SumDenOutMin=[]  SumDenOutMax=[]  SumNumOutMin=[]  SumNumOutMax=[]  DivideOutMin=[]  DivideOutMax=[]  UdiffTsProdOutMin=[]  UdiffTsProdOutMax=[]  NTsProdOutMin=[]  NTsProdOutMax=[]  UintegralTsProdOutMin=[]  UintegralTsProdOutMax=[]  UngainTsProdOutMin=[]  UngainTsProdOutMax=[]  ClampingZeroOutDataTypeStr=Inherit: Inherit via back propagation  ClampingZeroOutMin=[]  ClampingZeroOutMax=[]  FilterDenConstantOutDataTypeStr=Inherit: Inherit via back propagation  FilterDenConstantOutMin=[]  FilterDenConstantOutMax=[]  PCopyOutDataTypeStr=Inherit: Inherit via back propagation  PCopyOutMin=[]  PCopyOutMax=[]  NCopyOutDataTypeStr=Inherit: Inherit via back propagation  NCopyOutMin=[]  NCopyOutMax=[]  IntegratorContinuousStateAttributes=''  IntegratorStateMustResolveToSignalObject=off  IntegratorRTWStateStorageClass=Auto  FilterContinuousStateAttributes=''  FilterStateMustResolveToSignalObject=off  FilterRTWStateStorageClass=Auto  ParallelPVariant=InternalParameters  IdealPVariant=Disabled  IVariant=InternalParameters  DVariant=InternalParameters  IntegratorVariant=Discrete  SatVariant=Enabled  AWVariant=DiscClampingParallel  PCopyVariant=Disabled  TRVariant=Disabled  FdbkBlocksVariant=Forward  IdealPFdbkVariant=Disabled  SatFdbkVariant=Disabled  DerivativeFilterVariant=ForwardEulerFilter  NVariant=InternalParameters  NCopyVariant=Disabled  FilterICVariant=InternalICsFilter  IntegratorICVariant=InternalICs  ExternalResetVariant=Disabled  TRSumVariant=Passthrough  SumFdbkVariant=Disabled  SumVariant=Sum_PID  TsampFilterVariant=InternalTs  TsampNgainVariant=Passthrough  TsampIntegralVariant=Disabled_SignalSpec  ExternalSaturationOutDataTypeStr=Inherit: Same as second input
  Accel Cmd : Outport
  wires:
  Velocity Cmd/1 -> Add/1
  UAV State/1 -> Bus Selector/1
  Bus Selector/1 -> Add/2  "<WorldVelocity>"
  Add/1 -> Demux/1
  Demux/1 -> PID Controller/1
  Demux/2 -> PID Controller1/1
  Demux/3 -> PID Controller2/1
  PID Controller/1 -> Mux/1
  PID Controller1/1 -> Mux/2
  PID Controller2/1 -> Mux/3
  Mux/1 -> Accel Cmd/1

== matlab function NIMBY/Obstacle Avoidance/MATLAB Function1 ==
  data: flag output; safeLAP output; LAP input; tpose input; Position input; Width input; Height input; escapeMargin input
%% Name: isRestricted
%  Author: Josh Josey
%  Purpose: Determines if the drone is in a restricted zone or plans to
%           path into one
%
%  Input:   LAP = the UAVs lookahead point
%           tpose = the UAVs current position
%           Position = Nx3 array containing the position of obstacles
%           Width = the width of the obstacles
%           Height = the height of the obstacles
%           escapeMargin = how far out the drone should path to esacpe an
%                          obstacle
%  Output:  flag = the flag signal, >=1 if it is restricted
%           safeLAP = a LAP that will avoid or escape restricted zones
function [flag,safeLAP] = isRestricted(LAP, tpose, Position, Width, Height, escapeMargin)
    %assume it is not restrictred
    safeLAP = LAP;
    flag = 0;

    %Check if the UAV is currently in a restricted zone
    for i = 1:size(Position,1)
        %check the x bounds
        if tpose(1) >  Position(i,1)-Width/2 && tpose(1) < Position(i,1)+ Width/2
            %check the y bounds
            if tpose(2) >  Position(i,2)- Width/2 && tpose(2) <  Position(i,2)+ Width/2
                %check the z bounds
                if abs(tpose(3)) >  Position(i,3) && abs(tpose(3)) <  Position(i,3)+ Height
                    %disp("Inside restricted zone");
                    %disp(i);
                    flag = 1;
                    %plan an escape
                    safeLAP = escapeFunction(tpose,Position(i,:),Width,escapeMargin);
                end
            end
        end
    end

    %if the path will pass through
    if flag ~= 1
        wp2 = LAP;
        wp1 = tpose;
        flag = 0;
        %generate Ax+By+C values
        A = wp2(2) - wp1(2);
        B = wp1(1) - wp2(1);
        C = wp2(1)*wp1(2) - wp1(1)*wp2(2);
        %test each restricted zone
        for i = 1:size(Position,1)
            %get the vertices
            v1 = [Position(i,1)-Width/2 Position(i,2)-Width/2];
            v2 = [Position(i,1)+Width/2 Position(i,2)-Width/2];
            v3 = [Position(i,1)+Width/2 Position(i,2)+Width/2];
            v4 = [Position(i,1)-Width/2 Position(i,2)+Width/2];
            vertices = [v1; v2; v3; v4; v1];
            %test each edge
            for j = 1:size(vertices,1)-1
                %test the position of the vertex 1 relative to the line
                test1 = A*vertices(j,1) + B*vertices(j,2) + C;
                %test the position of the vertex 2 relative to the line
                test2 = A*vertices(j+1,1) + B*vertices(j+1,2) + C;
                %if the signs are different, invasion will occur         
                if sign(test1) ~= sign(test2)
                    %fprintf("Invastion on obstacle %d at edge from V%d to V%d\n",i,j,j+1);
                    %disp("INVADE")
                    safeLAP = [tpose(1); tpose(2); tpose(3)];
                    flag = 1;
                    return
                end
            end
        end
    end
end

%% Name: escapeFunction
%  Author: Josh Josey
%  Purpose: Find the nearest edge out from a restricted zone and path to it
%  Input:   pose = the UAVs current position
%           obsPosition = Nx3 array containing the position of obstacles
%           obsWidth = the width of the obstacles
%           margin = how far out the drone should path to esacpe an
%                    obstacle
%  Output:   newPt = the escape waypoint
function newPt = escapeFunction(pose,obsPosition,obsWidth,margin)
    %Get the nearest boundary coordinates
    if pose(1) < obsPosition(1)
        x = obsPosition(1) - obsWidth/2 - margin; %-x direction
    else
        x = obsPosition(1) + obsWidth/2 + margin; %+x direction
    end

    if pose(2) < obsPosition(2)
        y = obsPosition(2) - obsWidth/2 - margin; %-y direction
    else
        y = obsPosition(2) + obsWidth/2 + margin; %+y direction
    end

    newPt = [x; y; pose(3)];
end

== matlab function NIMBY/MATLAB Function ==
  data: tpose input; x input; y input; z input; initialWPS input; restricted input; status input; out output; waypointLog output
%% Name: randomWaypoint
%  Author: Josh Josey
%  Purpose: Random waypoint mobility for the waypoint follower block
%  Input:    tpose = the UAVs current position
%            x,y,z = a random value for x,y,z respectively
%            initialWPS = a 2x3 array containing the initial position & wp
%            restricted = a flag denoting invasion into a restricted zone
%            status = the status of waypoint navigation, from the WP
%                       follower block
%  Output:   out = the [2x3] signal containing the waypoints
function [out,waypointLog]  = randomWaypoint(tpose,x,y,z,initialWPS, restricted, status)
    persistent nextWps
    distFlag = 0;
    waypointLog = [initialWPS(2,:)];
    %Check if the waypoints have been initialized
    if isempty(nextWps)
        nextWps = initialWPS;
    else
        %check the distance to the last waypoint
        dist = sqrt( (tpose(1) - nextWps(2,1))^2 + (tpose(2) - nextWps(2,2))^2 + (tpose(3) - nextWps(2,3))^2);
        if dist < 1
            distFlag = 1;
        end
    end
    
    %if the drone is within distance and all waypoint have been visited,
    if status == 1 && distFlag == 1
            %move to the next waypoint and log the previous   
            nextWps = [nextWps(2,:); x(1) y(1) -z(1)];
            %waypoints = [waypoints; x y -z];
            waypointLog = nextWps(2,:);
    end
    
    %if the drone is going to enter a restricted area
    if restricted == 1
        %disp("INVADE");
        nextWps = [x(1) y(1) -z(1); x(2) y(2) -z(2)];
    end
    
    %output the waypooints
    out = nextWps;
    
end

== matlab function NIMBY/Position, Velocity, Acceleration Control/Subsystem/Multirotor Acceleration Control ==
  data: acc input; roll output; pitch output; thrust output; yaw input; DroneMass parameter; Gravity parameter
%% accControl
% Author: Mathworks, Comments added by Josh Josey
% Purpose:  Converts the acceleration command into control values 
%           for roll, pitch, and thrust
%
%  Input:   acc = the acceleration command
%           yaw = the drone's current yaw
%           DroneMass = the drone's mass
%           Gravity = the value of gravity defined in the workspace
%
%  Output:  roll = the control signal for the roll
%           pitch = the control signal for the pitch
%           thrust = the control signal for the thrust
function [roll, pitch, thrust] = accControl(acc, yaw, DroneMass, Gravity)
    
    %get the x,y,z acceleration vectors
    xddot = acc(1);
    yddot = acc(2);
    zddot = acc(3);
    
    %calculate pitch based on the combined horizontal acceleration (x,y) and the
    %vertical acceleration (z) compensated with gravity
    pitch = atan2((-xddot*cos(yaw)-yddot*sin(yaw)), ( -zddot + Gravity));
    
    %calculate the roll based on the combination of the horizontal
    %acceleration (x,y) compensated for the yaw and pitch as well as the
    %vertical acceleration compensated with gravity
    roll = atan2(((-xddot*sin(yaw)+yddot*cos(yaw))*cos(pitch)), (-zddot+Gravity));
    
    %limit the roll and pitch to 25 degrees or 0.4 radians
    roll_limit = 25*pi/180;
    pitch_limit = 25*pi/180;
    
    %ensure the roll and pitch stay betweent the limits
    roll = min(roll_limit, max(-roll_limit, roll));
    pitch = min(pitch_limit, max(-pitch_limit, pitch));
    
    %calculate the thrust to achieve the desired vertical acceleration
    %using the current vertical acceleration and the pitch and roll
    thrust = DroneMass*(-zddot+Gravity)/(cos(pitch)*cos(roll));
end
